simulink model "propLisboa"  (Simulink 9.3)
settings: Solver=ode45  StartTime=0  StopTime=8760  RelTol=1e-1  EnableMultiTasking=on
PreLoadFcn:
  | A=[-0.0418]
  | 
  | B=[0.0214, 0.0204, 0.0013, 0.0012, 0.0011, 0.0011]
  | 
  | C=[0.0448; 0.0474]
  | 
  | D = [0.0448, 0.0474, 0.1029, 0.0499, 0, 0; 0.0027, 0.0029, 0.0056, 0.0027, 0.0056, 0.0027]
InitFcn:
  | K=1
settings Model: Creator=Administrator  LastModifiedBy=HP
settings SolverCC: MaxConsecutiveZCs=2000
settings DataIOCC: LimitDataPoints=on
settings OptimizationCC: ExpressionDepthLimit=2147483647  InitFltsAndDblsToZero=on
settings DebuggingCC: SaveWithParameterizedLinksMsg=none  SignalResolutionControl=TryResolveAllWithWarning  SolverPrmCheckMsg=warning  MultiTaskDSMMsg=warning  MultiTaskCondExecSysMsg=none  StateNameClashWarn=warning
settings GRTTargetCC: TargetFcnLib=ansi_tfl_tmw.mat  GeneratePreprocessorConditionals=Disable all

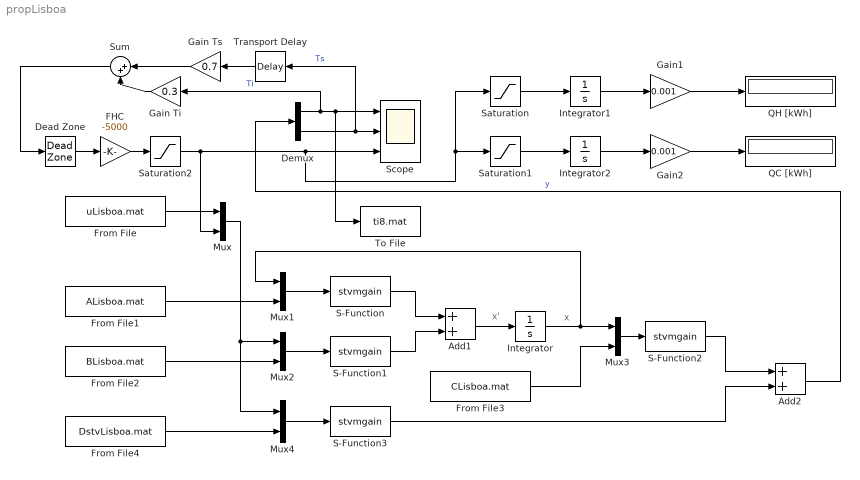
== system propLisboa ==
  note: x
  note: x'
  Add1 : Sum
  Add2 : Sum
  Dead Zone : DeadZone  LowerValue=20  UpperValue=26  ZeroCross=off  SaturateOnIntegerOverflow=on
  Demux : Demux  Outputs=2
  FHC : Gain  Gain=-5000
  From File : FromFile  FileName=uLisboa.mat  SampleTime=1
  From File1 : FromFile  FileName=ALisboa.mat  SampleTime=1
  From File2 : FromFile  FileName=BLisboa.mat  SampleTime=1
  From File3 : FromFile  FileName=CLisboa.mat  SampleTime=1
  From File4 : FromFile  FileName=DstvLisboa.mat  SampleTime=1
  Gain Ti : Gain  Gain=0.3
  Gain Ts : Gain  Gain=0.7
  Gain1 : Gain  Gain=0.001  SampleTime=1
  Gain2 : Gain  Gain=0.001  SampleTime=1
  Integrator : Integrator  InitialCondition=18
  Integrator1 : Integrator
  Integrator2 : Integrator
  Mux : Mux  Inputs=2
  Mux1 : Mux  Inputs=[1 1]
  Mux2 : Mux  Inputs=[6 6]
  Mux3 : Mux  Inputs=[1 2]
  Mux4 : Mux  Inputs=[6 12]
  QC [kWh] : Display
      settings: Format=bank  SampleTime=1
  QH [kWh] : Display
      settings: Format=bank  SampleTime=1
  S-Function : S-Function  FunctionName=stvmgain  Parameters=1, -1  SFunctionDeploymentMode=off  EnableBusSupport=off
  S-Function1 : S-Function  FunctionName=stvmgain  Parameters=[1 1 1 1 1 1], -1  SFunctionDeploymentMode=off  EnableBusSupport=off
  S-Function2 : S-Function  FunctionName=stvmgain  Parameters=[1 ;1] -1  SFunctionDeploymentMode=off  EnableBusSupport=off
  S-Function3 : S-Function  FunctionName=stvmgain  Parameters=[1 1 1 1 1 1; 1 1 1 1 1 1], -1  SFunctionDeploymentMode=off  EnableBusSupport=off
  Saturation : Saturate  UpperLimit=20000  LowerLimit=0  SampleTime=1
  Saturation1 : Saturate  UpperLimit=0  LowerLimit=-20000  SampleTime=1
  Saturation2 : Saturate  UpperLimit=10000  LowerLimit=-10000
  Scope : Scope  NumInputPorts=3
  Sum : Sum  Inputs=|++
  To File : ToFile  Filename=ti8.mat  SampleTime=1
  Transport Delay : TransportDelay
  wires:
  From File/1 -> Mux/1
  Demux/2 -> Scope/2, Transport Delay/1  "Ts"
  Demux/1 -> Gain Ti/1, Scope/1, To File/1  "Ti"
  From File1/1 -> Mux1/2
  Mux1/1 -> S-Function/1
  From File2/1 -> Mux2/2
  Mux/1 -> Mux2/1, Mux4/1
  Mux2/1 -> S-Function1/1
  S-Function/1 -> Add1/1
  S-Function1/1 -> Add1/2
  Add1/1 -> Integrator/1
  Integrator/1 -> Mux3/1, Mux1/1
  Mux3/1 -> S-Function2/1
  Mux4/1 -> S-Function3/1
  S-Function2/1 -> Add2/1
  S-Function3/1 -> Add2/2
  Add2/1 -> Demux/1  "y"
  From File4/1 -> Mux4/2
  From File3/1 -> Mux3/2
  Dead Zone/1 -> FHC/1
  FHC/1 -> Saturation2/1
  Integrator1/1 -> Gain1/1
  Gain1/1 -> QH [kWh]/1
  Integrator2/1 -> Gain2/1
  Saturation1/1 -> Integrator2/1
  Saturation/1 -> Integrator1/1
  Saturation2/1 -> Mux/2, Scope/3, Saturation1/1, Saturation/1
  Gain2/1 -> QC [kWh]/1
  Sum/1 -> Dead Zone/1
  Gain Ts/1 -> Sum/1
  Gain Ti/1 -> Sum/2
  Transport Delay/1 -> Gain Ts/1
